simulink model "Shanthan_Heeirthan_Hwk11_Q4R06"  (R2023a)
settings: Solver=FixedStepDiscrete  StartTime=0.0  StopTime=100  FixedStep=1/50  RelTol=1e-3
InitFcn:
  | % Set the current directory
  | cd(fileparts(which(bdroot)));
  | ShanthanHeeirthanFPscript4
values from neighbouring files (symbols this model uses):
  Denlpx = TFlpx.Den{1}    [ShanthanHeeirthanFPscript4.m]
  Denlpy = TFlpy.Den{1}    [ShanthanHeeirthanFPscript4.m]
  Denlpz = TFlpz.Den{1}    [ShanthanHeeirthanFPscript4.m]
  Numlpx = TFlpx.Num{1}    [ShanthanHeeirthanFPscript4.m]
  Numlpy = TFlpy.Num{1}    [ShanthanHeeirthanFPscript4.m]
  Numlpz = TFlpz.Num{1}    [ShanthanHeeirthanFPscript4.m]
undefined symbols (not defined in the file or in its folder): Fs
libraries: dspsigops x4, instrumentseriallib x3
settings Model: Creator=bruders  LastModifiedBy=shanthah
settings DataIOCC: ReturnWorkspaceOutputs=off
settings DebuggingCC: UnconnectedInputMsg=warning  UnconnectedOutputMsg=warning  UnconnectedLineMsg=warning
settings ModelReferenceCC: EnableRefExpFcnMdlSchedulingChecks=on
settings RTWCC: DLArmComputeVersion=19.05

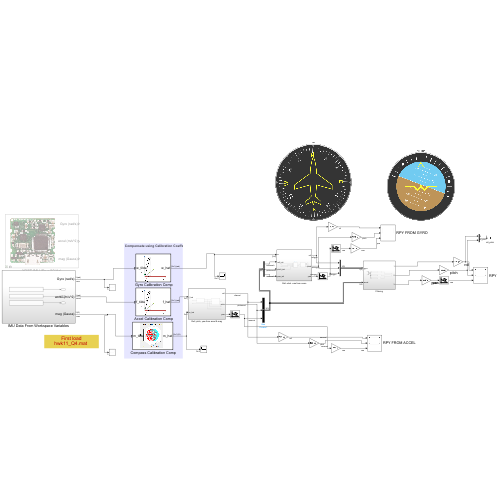
[thumbnail: Simulink's stored preview of the top-level diagram]
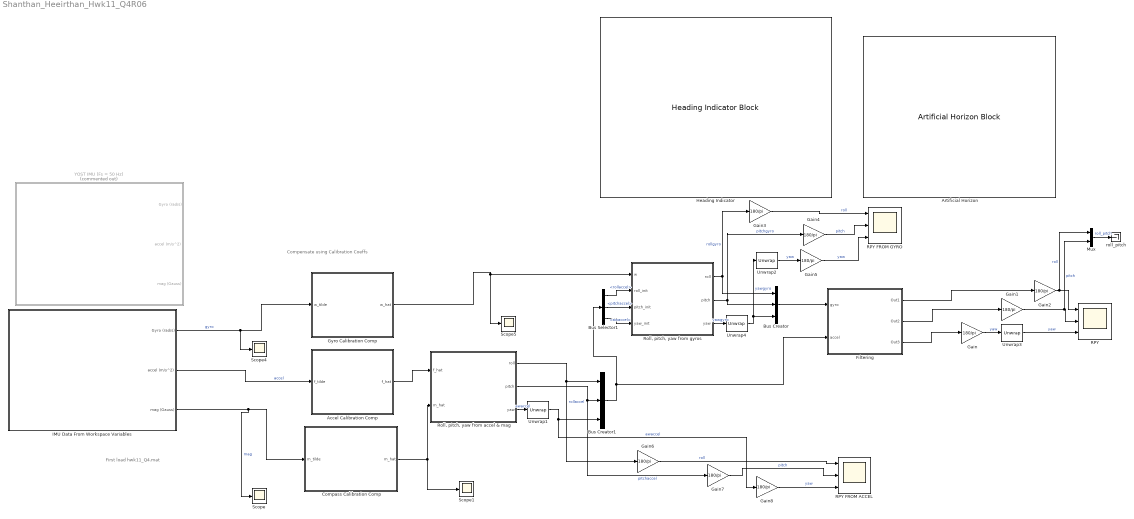
== system Shanthan_Heeirthan_Hwk11_Q4R06 ==
  note: Compensate using Calibration Coeffs
  note: First load hwk11_Q4.mat
  " Accel Calibration Comp" : MATLAB Function  TreatAsAtomicUnit=on
  " Compass Calibration Comp" : MATLAB Function  TreatAsAtomicUnit=on
  " Gyro Calibration Comp" : MATLAB Function  TreatAsAtomicUnit=on
  Artificial Horizon : ArtificialHorizonBlock
  Bus Creator : BusCreator  Inputs=3
  Bus Creator1 : BusCreator  Inputs=3
  Bus Selector1 : BusSelector  OutputSignals=rollaccel,pitchaccel,awaccel
  Filtering : Subsystem
  Gain{,1..8} (9 alike) : Gain  Gain=180/pi
  Heading Indicator : HeadingIndicatorBlock
  IMU Data From Workspace Variables : Subsystem
  Mux : Mux  Inputs=2
  "RPY " : Scope  NumInputPorts=3
  RPY FROM ACCEL : Scope  NumInputPorts=3
  RPY FROM GYRO : Scope  NumInputPorts=3
  "Roll, pitch, yaw from accel & mag" : Subsystem
  "Roll, pitch, yaw from gyros" : Subsystem
  Scope{,1,4..5} (4 alike) : Scope
  Unwrap{1..4} (4 alike) : dspsigops/Unwrap  tol=pi  InputProcessing=Columns as channels (frame based)  running=off
  YOST IMU (Fs = 50 Hz) : Subsystem  Commented=on  InitFcn=|
      | % Determine the available serial ports
      | comPort = serialportlist("available");
      | 
      | % Assume that the last serial port added is the IMU
      | MyComPort = comPort(end);
      | 
      | % Get the name of the current Simulink file
      | fn = gcs;
      | 
      | % Set the COM port of the IMU in three blocks
      | set_param([fn, '/YOST IMU (Fs = 50 Hz)/Serial Configuration'],'Port', MyComPort)
      | set_param([fn, '/YOST IMU (Fs = 50 Hz)/Serial Receive'],'Port', MyComPort)
      | set_param([fn, '/YOST IMU (Fs = 50 Hz)/Initialize Function/Serial Send'],'Port', MyComPort)
      mask Display: image('$imagefile'); % Use "Edit Image" on toolstrip to change.
  roll_pitch : Terminator
  wires:
  " Gyro Calibration Comp"/1(w_hat) -> "Roll, pitch, yaw from gyros"/1(w), Scope5/1
  " Accel Calibration Comp"/1(f_hat) -> "Roll, pitch, yaw from accel & mag"/1(f_hat)
  " Compass Calibration Comp"/1(m_hat) -> "Roll, pitch, yaw from accel & mag"/2(m_hat), Scope1/1
  Gain2/1 -> Mux/1, "RPY "/1  "roll"
  Gain/1 -> Unwrap3/1  "yaw"
  Gain1/1 -> Mux/2, "RPY "/2  "pitch"
  IMU Data From Workspace Variables/1(Gyro (rad/s)) -> " Gyro Calibration Comp"/1(w_tilde), Scope4/1  "gyro"
  IMU Data From Workspace Variables/2(accel (m/s^2)) -> " Accel Calibration Comp"/1(f_tilde)  "accel"
  IMU Data From Workspace Variables/3(mag (Gauss)) -> Scope/1, " Compass Calibration Comp"/1(m_tilde)  "mag"
  "Roll, pitch, yaw from gyros"/1(roll) -> Bus Creator/1, Gain3/1  "rollgyro"
  "Roll, pitch, yaw from gyros"/2(pitch) -> Bus Creator/2, Gain4/1  "pitchgyro"
  "Roll, pitch, yaw from gyros"/3(yaw) -> Unwrap4/1  "yawgyro"
  "Roll, pitch, yaw from accel & mag"/1(roll) -> Gain6/1, Bus Creator1/1  "rollaccel"
  "Roll, pitch, yaw from accel & mag"/2(pitch) -> Gain7/1, Bus Creator1/2  "pitchaccel"
  "Roll, pitch, yaw from accel & mag"/3(yaw) -> Unwrap1/1  "awaccel"
  Bus Creator1/1 -> Bus Selector1/1, Filtering/2(accel)
  Bus Selector1/1 -> "Roll, pitch, yaw from gyros"/2(roll_init)  "<rollaccel>"
  Bus Selector1/2 -> "Roll, pitch, yaw from gyros"/3(pitch_init)  "<pitchaccel>"
  Bus Selector1/3 -> "Roll, pitch, yaw from gyros"/4(yaw_init)  "<awaccel>"
  Filtering/1(Out1) -> Gain2/1
  Filtering/2(Out2) -> Gain1/1
  Bus Creator/1 -> Filtering/1(gyro)
  Mux/1 -> roll_pitch/1  "roll_pitch"
  Gain3/1 -> RPY FROM GYRO/1  "roll"
  Gain4/1 -> RPY FROM GYRO/2  "pitch"
  Gain5/1 -> RPY FROM GYRO/3  "yaw"
  Gain6/1 -> RPY FROM ACCEL/1  "roll"
  Gain7/1 -> RPY FROM ACCEL/2  "pitch"
  Gain8/1 -> RPY FROM ACCEL/3  "yaw"
  Unwrap2/1 -> Gain5/1  "yaw"
  Filtering/3(Out3) -> Gain/1
  Unwrap3/1 -> "RPY "/3  "yaw"
  Unwrap1/1 -> Gain8/1, Bus Creator1/3  "awaccel"
  Unwrap4/1 -> Bus Creator/3, Unwrap2/1  "yawgyro"

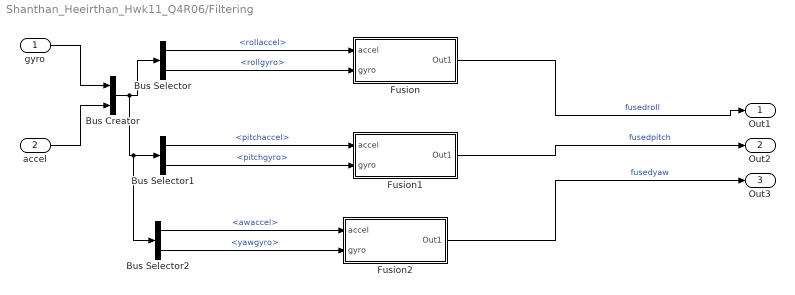
== system Shanthan_Heeirthan_Hwk11_Q4R06/Filtering ==
  gyro : Inport
  accel : Inport  Port=2
  Bus Creator : BusCreator  Inputs=2
  Bus Selector : BusSelector  OutputSignals=signal2.rollaccel,signal1.rollgyro
  Bus Selector1 : BusSelector  OutputSignals=signal2.pitchaccel,signal1.pitchgyro
  Bus Selector2 : BusSelector  OutputSignals=signal2.awaccel,signal1.yawgyro
  Fusion : Subsystem
  Fusion1 : Subsystem
  Fusion2 : Subsystem
  Out1 : Outport
  Out2 : Outport  Port=2
  Out3 : Outport  Port=3
  wires:
  gyro/1 -> Bus Creator/1
  accel/1 -> Bus Creator/2
  Bus Creator/1 -> Bus Selector2/1, Bus Selector1/1, Bus Selector/1
  Bus Selector/1 -> Fusion/1(accel)  "<rollaccel>"
  Bus Selector/2 -> Fusion/2(gyro)  "<rollgyro>"
  Fusion/1(Out1) -> Out1/1  "fusedroll"
  Bus Selector1/1 -> Fusion1/1(accel)  "<pitchaccel>"
  Bus Selector1/2 -> Fusion1/2(gyro)  "<pitchgyro>"
  Bus Selector2/1 -> Fusion2/1(accel)  "<awaccel>"
  Bus Selector2/2 -> Fusion2/2(gyro)  "<yawgyro>"
  Fusion1/1(Out1) -> Out2/1  "fusedpitch"
  Fusion2/1(Out1) -> Out3/1  "fusedyaw"

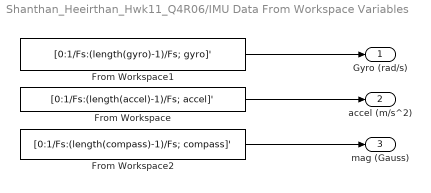
== system Shanthan_Heeirthan_Hwk11_Q4R06/IMU Data From Workspace Variables ==
  From Workspace : FromWorkspace  VariableName=[0:1/Fs:(length(accel)-1)/Fs; accel]'  SampleTime=1/Fs
  From Workspace1 : FromWorkspace  VariableName=[0:1/Fs:(length(gyro)-1)/Fs; gyro]'  SampleTime=1/Fs
  From Workspace2 : FromWorkspace  VariableName=[0:1/Fs:(length(compass)-1)/Fs; compass]'  SampleTime=1/Fs
  Gyro (rad/s) : Outport
  accel (m/s^2) : Outport  Port=2
  mag (Gauss) : Outport  Port=3
  wires:
  From Workspace/1 -> accel (m/s^2)/1
  From Workspace1/1 -> Gyro (rad/s)/1
  From Workspace2/1 -> mag (Gauss)/1

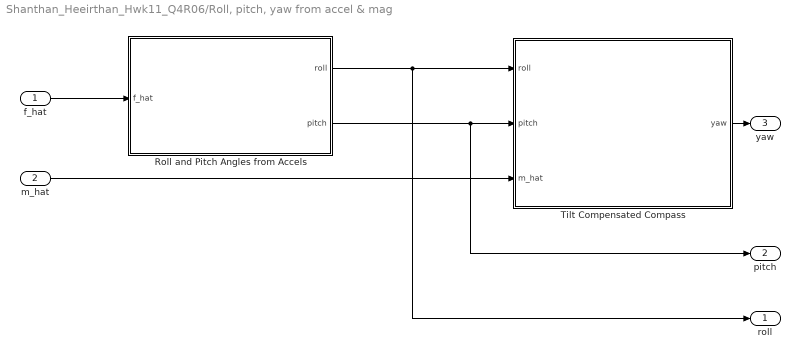
== system Shanthan_Heeirthan_Hwk11_Q4R06/Roll, pitch, yaw from accel & mag ==
  f_hat : Inport
  m_hat : Inport  Port=2
  Roll and Pitch Angles from Accels : MATLAB Function  TreatAsAtomicUnit=on
  Tilt Compensated Compass : MATLAB Function  TreatAsAtomicUnit=on
  roll : Outport
  pitch : Outport  Port=2
  yaw : Outport  Port=3
  wires:
  Roll and Pitch Angles from Accels/2(pitch) -> pitch/1, Tilt Compensated Compass/2(pitch)
  Tilt Compensated Compass/1(yaw) -> yaw/1
  Roll and Pitch Angles from Accels/1(roll) -> roll/1, Tilt Compensated Compass/1(roll)
  m_hat/1 -> Tilt Compensated Compass/3(m_hat)
  f_hat/1 -> Roll and Pitch Angles from Accels/1(f_hat)

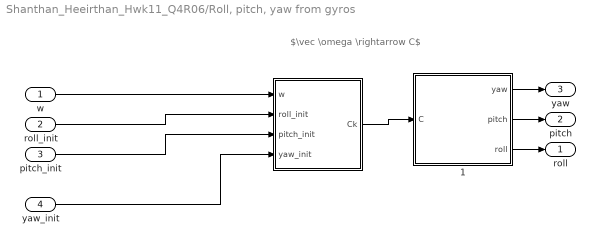
== system Shanthan_Heeirthan_Hwk11_Q4R06/Roll, pitch, yaw from gyros ==
  note: $\vec \omega \rightarrow C$
  w : Inport
  roll_init : Inport  Port=2
  pitch_init : Inport  Port=3
  yaw_init : Inport  Port=4
  " " : MATLAB Function  TreatAsAtomicUnit=on
  " 1" : MATLAB Function  TreatAsAtomicUnit=on
  roll : Outport
  pitch : Outport  Port=2
  yaw : Outport  Port=3
  wires:
  " "/1(Ck) -> " 1"/1(C)
  w/1 -> " "/1(w)
  " 1"/1(yaw) -> yaw/1
  " 1"/2(pitch) -> pitch/1
  " 1"/3(roll) -> roll/1
  roll_init/1 -> " "/2(roll_init)
  pitch_init/1 -> " "/3(pitch_init)
  yaw_init/1 -> " "/4(yaw_init)

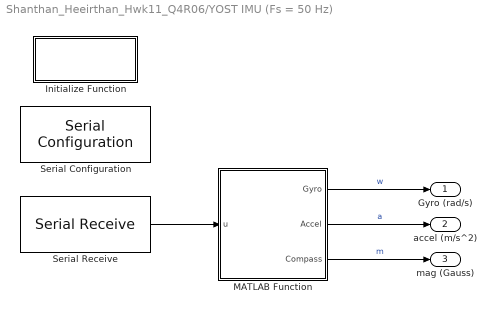
== system Shanthan_Heeirthan_Hwk11_Q4R06/YOST IMU (Fs = 50 Hz) ==
  Initialize Function : Subsystem  TreatAsAtomicUnit=on
  MATLAB Function : MATLAB Function  TreatAsAtomicUnit=on
  Serial Configuration : instrumentseriallib/Serial Configuration  Priority=-200000  PortSel=COM5  Port=COM5  ComPort=COM5  BaudRate=115200  DataBits=8  Parity=none  StopBits=1  ByteOrder=big-endian  FlowControl=none  Timeout=2  SimulateUsing=Interpreted execution  BlockInModel=on  aMode=1
  Serial Receive : instrumentseriallib/Serial Receive  Priority=1  PortSel=COM5  Port=COM5  ComPort=COM5  DataType=uint8  SaveDataType=uint8  ToggleHeader=off  Header=[]  ToggleTerminator=on  Terminator=<none>  CustomTerminator=[]  InputFormat=Row major  ToggleDataSize=on  DataSize=[1 36]  EnableBlockingMode=on  ActionDataUnavailable=Output custom value  ActionWhenDataUnavailable=Output custom value  CustomValue=9  SampleTime=0.02  SimulateUsing=Interpreted execution  BlockInModel=on  aMode=1
  Gyro (rad/s) : Outport
  accel (m/s^2) : Outport  Port=2
  mag (Gauss) : Outport  Port=3
  wires:
  Serial Receive/1 -> MATLAB Function/1(u)
  MATLAB Function/2(Accel) -> accel (m/s^2)/1  "a"
  MATLAB Function/1(Gyro) -> Gyro (rad/s)/1  "w"
  MATLAB Function/3(Compass) -> mag (Gauss)/1  "m"

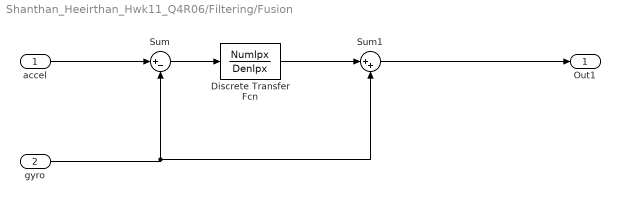
== system Shanthan_Heeirthan_Hwk11_Q4R06/Filtering/Fusion ==
  accel : Inport
  gyro : Inport  Port=2
  Discrete Transfer Fcn : DiscreteTransferFcn  Numerator=Numlpx  Denominator=Denlpx  SampleTime=.02
  Sum : Sum  Inputs=|+-
  Sum1 : Sum  Inputs=|++
  Out1 : Outport
  wires:
  accel/1 -> Sum/1
  Sum/1 -> Discrete Transfer Fcn/1
  Discrete Transfer Fcn/1 -> Sum1/1
  gyro/1 -> Sum1/2, Sum/2
  Sum1/1 -> Out1/1

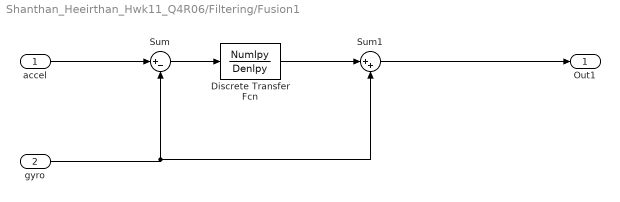
== system Shanthan_Heeirthan_Hwk11_Q4R06/Filtering/Fusion1 ==
  accel : Inport
  gyro : Inport  Port=2
  Discrete Transfer Fcn : DiscreteTransferFcn  Numerator=Numlpy  Denominator=Denlpy  SampleTime=0.02
  Sum : Sum  Inputs=|+-
  Sum1 : Sum  Inputs=|++
  Out1 : Outport
  wires:
  accel/1 -> Sum/1
  Sum/1 -> Discrete Transfer Fcn/1
  Discrete Transfer Fcn/1 -> Sum1/1
  gyro/1 -> Sum1/2, Sum/2
  Sum1/1 -> Out1/1

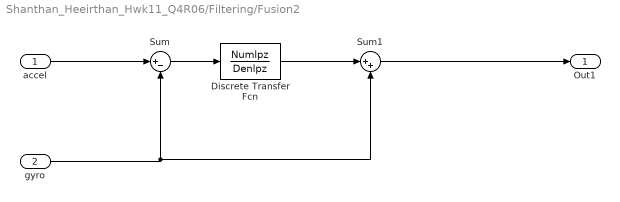
== system Shanthan_Heeirthan_Hwk11_Q4R06/Filtering/Fusion2 ==
  accel : Inport
  gyro : Inport  Port=2
  Discrete Transfer Fcn : DiscreteTransferFcn  Numerator=Numlpz  Denominator=Denlpz  SampleTime=0.02
  Sum : Sum  Inputs=|+-
  Sum1 : Sum  Inputs=|++
  Out1 : Outport
  wires:
  accel/1 -> Sum/1
  Sum/1 -> Discrete Transfer Fcn/1
  Discrete Transfer Fcn/1 -> Sum1/1
  gyro/1 -> Sum1/2, Sum/2
  Sum1/1 -> Out1/1

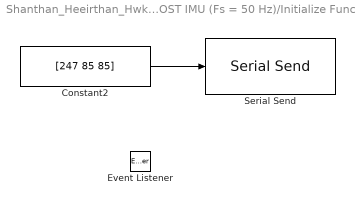
== system Shanthan_Heeirthan_Hwk11_Q4R06/YOST IMU (Fs = 50 Hz)/Initialize Function ==
  Constant2 : Constant  Value=[247 85 85]  OutDataTypeStr=uint8  SampleTime=-1
  Event Listener : EventListener  DisableCoverage=on  EventName=reset
  Serial Send : instrumentseriallib/Serial Send  Priority=1  PortSel=COM5  Port=COM5  ComPort=COM5  Header=[]  Terminator=<none>  CustomTerminator=[]  EnableBlockingMode=on  SimulateUsing=Interpreted execution  BlockInModel=on  aMode=1
  wires:
  Constant2/1 -> Serial Send/1

== matlab function Shanthan_Heeirthan_Hwk11_Q4R06/Roll, pitch, yaw from gyros/  ==
  data: w input; Ck output; roll_init input; pitch_init input; yaw_init input
function Ck  = w2Cmat(w,roll_init,pitch_init,yaw_init)
% Description:
%   Computes attitude/orientation as a rotation matrix (C) from angular
%   velocity (w)
%
% Input:
%   w - Angular velocity at time t_k (rad/s)
%
% Output:
%   Ck - Attitude/orientation as a rotation matrix (C) at time t_k
%
% NOTE(s):
%   By default the attitude is initialized as an identity matrix

persistent Ck_1 Fs dt   % Attitude at time t_(k - 1)
if isempty(Ck_1)        % If the first call initialize the attitude
   %Ck_1 = ypr2dcm(yaw_init,pitch_init,roll_init);      % Initial attitude/orientation
   Ck_1 = eye(3); 
   Fs = 50;            % Sample frequency (Hz)
    dt = 1 / Fs;        % Sample interval (sec)
end

% Step 1: Compute the angle and axis of rotation
    theta_dot = norm(w);       % Angular speed (rad/s)n
    theta = theta_dot*dt;         % Angle rotated from time t(k-1) to t(k)
    k = w/norm(w);              % k = Normalized Axis of rotation

% Step 2: Compute the "small" change of attitude (i.e., Delta_C) over time dT
    K = [ 0 -k(3) k(2)         % Axis of rotation as a skew-symmetric matrix (dimless)
          k(3) 0 -k(1) 
          -k(2) k(1) 0 ];
 
    Delta_C = eye(3) + sin(theta) * K + (1-cos(theta)) * K^2; % Rodrigues Formula

% Step 3: Update the attitude: C(k-1) -> C(k)
    Ck = Ck_1*Delta_C;  % Fixed or relative axis rotation?

Ck_1 = Ck;              % Store the current attitude to use in the next sample interval
end     % End of function

== matlab function Shanthan_Heeirthan_Hwk11_Q4R06/YOST IMU (Fs = 50 Hz)/MATLAB Function ==
  data: u input; Gyro output size=[3 1]; Accel output size=[3 1]; Compass output size=[3 1]
function [Gyro, Accel, Compass] = fcn(u)

% Function Description:
%   Reads one frame of the YOST IMU binary data from the serial port
%
% INPUTS:
%   u = Serial port object
%   
% OUTPUTS:
%   Gyro    3x1 Gyroscope triad (rad/s)
%   Accel   3x1 Accelerometer triad (m/s^2)
%   Compass 3x1 Magnetic Field (Gauss)

g = 9.8;                        % Approx accel due to gravity (m/s^2)

% Returns 36 bytes: Gyro 3X(4-bytes), Accel 3X(4-bytes), and Mag 3X(4-bytes)
    IMU_Data = swapbytes(typecast(uint8(u),'single'));  % Big-Endian
    IMU_Data = double(IMU_Data);
    
    Gyro     = IMU_Data(1:3)';       % 3x1 Gyro data (in rad/s)
    Accel    = IMU_Data(4:6)'*g;     % 3x1 Accel data array (in m/s^2)
    Compass  = IMU_Data(7:9)';       % 3x1 Compass data (in Gauss)
end

== matlab function Shanthan_Heeirthan_Hwk11_Q4R06/ Accel Calibration Comp ==
  data: f_tilde input size=[3 1]; f_hat output size=[3 1]
function f_hat   = Accel_Cal_Comp(f_tilde)
% Description:
%   Compensates for fixed-bias, scale factor, and misalignment errors
%   determined via rate-table calibration.
%
% Input:
%   f_tilde - Uncalibrated Accel specific force 3x1 vector (m/s^2)
%
% Output:
%   f_hat - Calibrated Accel specific force 3x1 vector (m/s^2)
%
% NOTE(s):
%   Uses the accel fixed bias b_FBa and misalignment matrix Ma to 
%   compensate for calibration errors
%
%  Reference:  
%   EE 440 Lecture notes: AHRS lecture 16 and hwk 6
g = 9.79193;
%accel = load('accel_cal_params_1700023D.mat');
Ma = [-0.0054 0.0122 -0.0164;
    -0.0120 -0.0074 0.0127;
    0.0174 -0.0076 -0.0054];    % Accel misalignment: A 3X3 matrix
b_FBa = [-0.0683 % Accel fixed bias: A 3X1 vector
        0.0298
        -0.0351];
%f_hat = f_tilde;
f_hat = (inv(eye(3)+Ma)*(f_tilde-b_FBa));   % Compensate the uncalibrated to yield calibrated
end     % End of function

== matlab function Shanthan_Heeirthan_Hwk11_Q4R06/ Compass Calibration Comp ==
  data: m_tilde input size=[3 1]; m_hat output size=[3 1]
function m_hat   = Compass_Cal_Comp(m_tilde)
% Description:
%   Compensates for fixed-bias and scale factor errors determined via 
%   2D or 3D (sphere or ellipsoid fit) compass calibration.
%
% Input:
%   m_tilde - Uncalibrated magnetic field 3x1 vector (Gauss)
%
% Output:
%   m_hat - Calibrated magnetic field 3x1 vector (Gauss)
%
% NOTE(s):
%   Uses the compass fixed bias b_FBc and misalignment matrix
%   Mc to compensate for calibration errors
%
%  Reference:  
%   EE 440 Lecture notes: AHRS lecture 18

%Mc = [1.0025 0 0;
%    0 1.0025 0;
%    0 0 1.0025];    % Compass scale factor (scalar or diagonal 3x3 matrix)
Mc = 1.0025;
b_FBc = [-0.0225 % Compass fixed bias: 3X1 vector
        0.0037
        -0.0337];
% 
% Mc = 0.0206;
% b_FBc = [-0.0077; 0.0197; -0.1481];
%m_hat = inv(eye(3)+Mc)*(m_tilde-b_FBc);    % Compensate the uncalibrated to yield calibrated
m_hat = (m_tilde-b_FBc)/Mc;
%m_hat = m_tilde;
end     % End of function

== matlab function Shanthan_Heeirthan_Hwk11_Q4R06/ Gyro Calibration Comp ==
  data: w_tilde input size=[3 1]; w_hat output size=[3 1]
function w_hat   = Gyro_Cal_Comp(w_tilde)
% Description:
%   Compensates for fixed-bias, scale factor, and misalignment errors
%   determined via rate-table calibration.
%
% Input:
%   w_tilde - Uncalibrated Gyro angular velocity 3x1 vector (rad/s)
%
% Output:
%   w_hat - Calibrated Gyro angular velocity 3x1 vector (rad/s)
%
% NOTE(s):
%   Uses the gyro fixed bias b_FBg and misalignment matrix Mg to 
%   compensate for calibration errors
%
%  Reference:  
%   EE 440 Lecture notes: AHRS lecture 16 and hwk 6
%gyro = load('gyro_cal_params_1700023D.mat');
Mg = [-0.0014 0.0065 -0.0146;
     -0.0051 -0.022 0.0047;
     0.0156 -0.0049 -0.0055];    % Gyro misalignment: A 3X3 matrix
b_FBg = [0.0024 % Gyro fixed bias: A 3X1 vector
         0.0107
         -0.0046];

w_hat = inv(eye(3)+Mg)*(w_tilde-b_FBg) ;   % Compensate the uncalibrated to yield calibrated
%w_hat = w_tilde;
end     % End of function

== matlab function Shanthan_Heeirthan_Hwk11_Q4R06/Roll, pitch, yaw from gyros/ 1 ==
  data: C input; yaw output; pitch output; roll output
function [yaw, pitch, roll] = dcm2ypr(C)
% Function Description:
%   Based on a relative-axis yaw, then pitch, then roll rotation sequence 
%   3X3 DCM matrix C = Rz(yaw) Ry(pitch) Rx(roll).  
%   This function accepts C and returns yaw, pitch, and roll angles
%
% INPUTS:
%   C = 3x3 direction cosine matrix (i.e., rotation matrix)
%   
% OUTPUTS:
%   yaw   = Initial rotation about the common z-axis (rad)
%   pitch = rotation about the new y-axis (rad)
%   roll  = rotation about the new x-axis (rad)
%
% Reference:
%   EE 440 lecture 4 slide 13

pitch = atan2(-C(3,1), sqrt(C(2,1)^2+C(1,1)^2));    % Pitch angle (rad)
% If Pitch not equal to ±90° (yaw and roll are undefined if Pitch = ±90°)
if abs(abs(pitch) - pi/2) > eps
    roll  = atan2( C(3,2),C(3,3));                  % Roll angle (rad)
    yaw   = atan2( C(2,1),C(1,1));                  % Yaw angle (rad)
else
   error('pitch is ±90° => yaw and roll are undefined!!');
end

end % Close function

== matlab function Shanthan_Heeirthan_Hwk11_Q4R06/Roll, pitch, yaw from accel & mag/Tilt Compensated Compass ==
  data: roll input; pitch input; m_hat input; yaw output
function yaw  = AHRS(roll, pitch, m_hat)
% FUNCTION DESCRIPTION:
%   Implements a tilt compensated compass to estimate yaw
%
% INPUTS:
%   roll  - Roll angle (rad)
%   pitch - Pitch angle (rad)
%   m_hat - Calibrated magnetic field 3x1 vector (Gauss)
%
% OUTPUTS:
%  yaw    - Yaw (i.e., heading)) angle (rad)
%
%  Reference:  
%   EE 440 Lecture notes: lecture 18

Declination = 10.6* pi/180;    % Approx declination angle in Prescott, AZ (rad)

mx = m_hat(1);      % Extract the x, y, and z scalar components of mag meas (T)
my = m_hat(2);
mz = m_hat(3);

mxll = cos(pitch)*mx + cos(roll)*mz*sin(pitch) + my*sin(pitch)*sin(roll);
myll = cos(roll)*my - mz*sin(roll);        
%yaw = atan2(-myll,mxll) + Declination;  % Compute yaw or heading (to True North)
yaw = atan2(-(cos(roll)*my-mz*sin(roll)),cos(pitch)*mx+cos(roll)*mz*sin(pitch)+my*sin(pitch)*sin(roll)) + Declination;
end     % End of function

== matlab function Shanthan_Heeirthan_Hwk11_Q4R06/Roll, pitch, yaw from accel & mag/Roll and Pitch Angles from Accels ==
  data: f_hat input; roll output; pitch output
function [roll, pitch] = Accel2RollPitch(f_hat)
% FUNCTION DESCRIPTION:
%   Estimate roll and pitch angles from STATIONARY accels
%
% INPUTS:
%   f_hat - Calibrated Accel specific force 3x1 vector (m/s^2)
%
% OUTPUTS:
%  roll     Roll angle (rad)
%  pitch    Pitch angle (rad)
%
%  Reference:  
%   EE 440 Lecture notes: AHRS lecture 17

fx = f_hat(1);      % Extract the x, y, and z scalar components of accel meas (m/s^2)
fy = f_hat(2);
fz = f_hat(3);

roll  = atan2(-fy,-fz);                % phi (rad)
pitch = atan2(fx,sqrt(fy^2+fz^2));  % theta (rad)

end     % End of function
